simulink model "PD_Controller"  (R2021a)
settings: Solver=VariableStepAuto  StartTime=0.0  StopTime=1  RelTol=1e-3
settings Model: Creator=Zicx  LastModifiedBy=Zicx
settings DataIOCC: SaveOutput=off  SaveTime=off

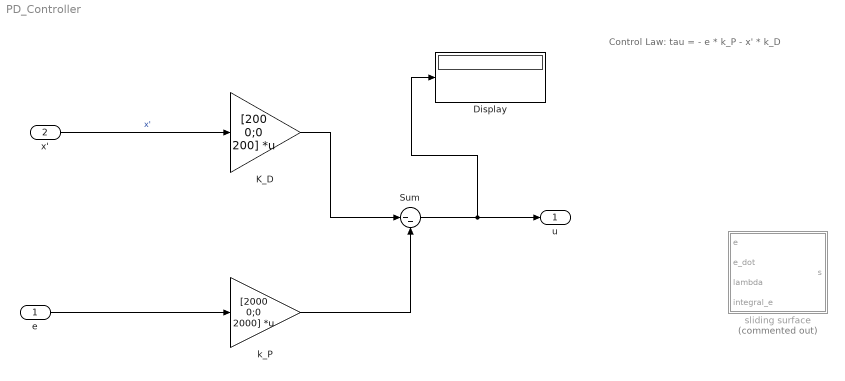
== system PD_Controller ==
  note: Control Law:
      |
      | tau = - e * k_P - x' * k_D
  e : Inport  OutDataTypeStr=double  PortDimensions=2  SampleTime=0
  x' : Inport  Port=2  OutDataTypeStr=double  PortDimensions=2  SampleTime=0
  Display : Display
  K_D : Gain  Gain=[200 0;0 200]  Multiplication=Matrix(K*u) (u vector)
  Sum : Sum  Inputs=|--
  k_P : Gain  Gain=[2000 0;0 2000]  Multiplication=Matrix(K*u) (u vector)
  sliding surface : MATLAB Function  Commented=on  TreatAsAtomicUnit=on
  u : Outport  OutDataTypeStr=double  PortDimensions=2  SampleTime=0
  wires:
  e/1 -> k_P/1
  K_D/1 -> Sum/1
  k_P/1 -> Sum/2
  Sum/1 -> u/1, Display/1
  x'/1 -> K_D/1  "x'"

== matlab function PD_Controller/sliding surface ==
  data: e input; s output; e_dot input; lambda input; integral_e input
function s = fcn(e, e_dot, lambda, integral_e)

s = e_dot + 2 * lambda * e + (lambda^2) * integral_e;
